simulink model "Hardware_Luo_Converter_with_IGBT"  (R2025a)
settings: Solver=VariableStepAuto  StartTime=0.0  StopTime=1  RelTol=1e-3
libraries: spsSeriesRLCBranchLib x5, spsMeanLib x5, spsCurrentMeasurementLib x2, spsVoltageMeasurementLib x2, spsDCVoltageSourceLib x1, spsDiodeLib x1, spsIGBTDiodeLib x1, sps_lib x1
settings Model: Creator=sanat  LastModifiedBy=sanat

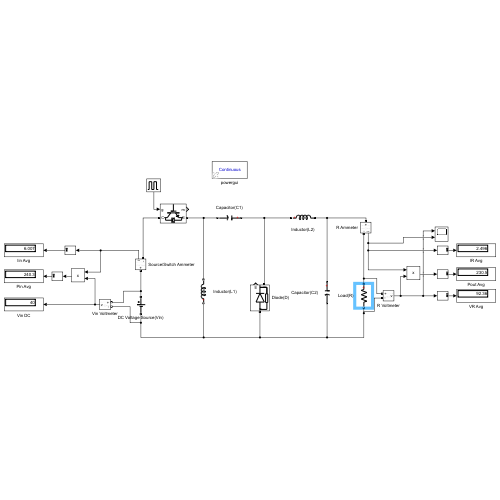
[thumbnail: Simulink's stored preview of the top-level diagram]
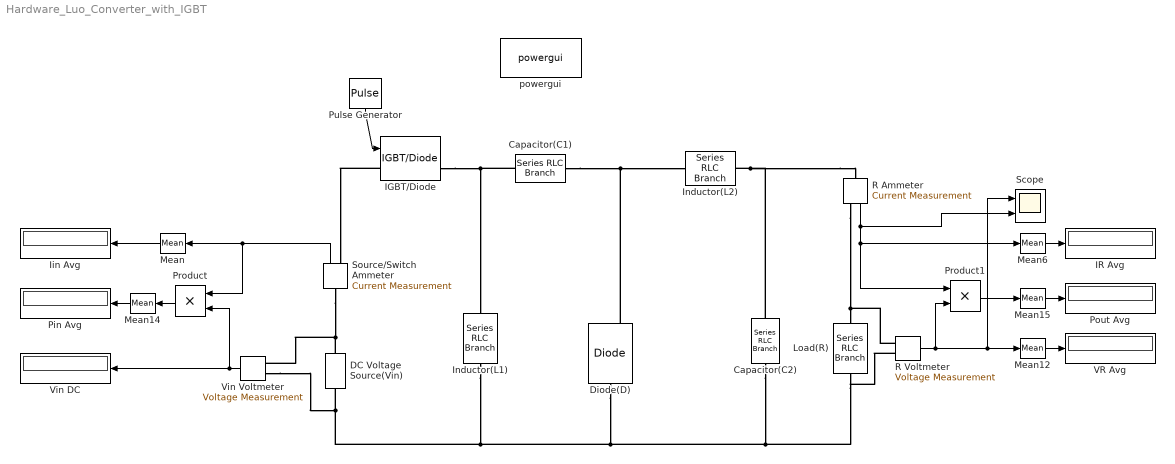
== system Hardware_Luo_Converter_with_IGBT ==
  Capacitor(C1) : spsSeriesRLCBranchLib/Series RLC Branch  LConnTagsString=__new0  RConnTagsString=__new0  BranchType=C  Resistance=1  Inductance=1e-3  SetiL0=off  InitialCurrent=0  Capacitance=470e-6  Setx0=off  InitialVoltage=0  Measurements=None
  Capacitor(C2) : spsSeriesRLCBranchLib/Series RLC Branch  LConnTagsString=__new0  RConnTagsString=__new0  BranchType=C  Resistance=1  Inductance=1e-3  SetiL0=off  InitialCurrent=0  Capacitance=470e-6  Setx0=off  InitialVoltage=0  Measurements=None
  DC Voltage Source(Vin) : spsDCVoltageSourceLib/DC Voltage Source  Amplitude=40  Measurements=None
  Diode(D) : spsDiodeLib/Diode  Ron=0.001  Lon=0  Vf=0.8  IC=0  UseSnubber=0  Rs=500  Cs=250e-9  Measurements=on
  IGBT/Diode : spsIGBTDiodeLib/IGBT//Diode  Ron=1e-2  Rs=1e5  Cs=inf  Measurements=on
  IR Avg : Display
  Iin Avg : Display
  Inductor(L1) : spsSeriesRLCBranchLib/Series RLC Branch  LConnTagsString=__new0  RConnTagsString=__new0  BranchType=L  Resistance=1  Inductance=3.32e-3  SetiL0=off  InitialCurrent=0  Capacitance=1e-6  Setx0=off  InitialVoltage=0  Measurements=None
  Inductor(L2) : spsSeriesRLCBranchLib/Series RLC Branch  LConnTagsString=__new0  RConnTagsString=__new0  BranchType=L  Resistance=1  Inductance=1.52e-3  SetiL0=off  InitialCurrent=0  Capacitance=1e-6  Setx0=off  InitialVoltage=0  Measurements=None
  Load(R) : spsSeriesRLCBranchLib/Series RLC Branch  LConnTagsString=__new0  RConnTagsString=__new0  BranchType=R  Resistance=37  Inductance=1e-3  SetiL0=off  InitialCurrent=0  Capacitance=1e-6  Setx0=off  InitialVoltage=0  Measurements=None
  Mean{,6,12,14..15} (5 alike) : spsMeanLib/Mean  Freq=60  Vinit=0  Ts=0
  Pin Avg : Display
  Pout Avg : Display
  Product : Product
  Product1 : Product
  Pulse Generator : DiscretePulseGenerator  PulseType=Time based  Period=1/20000  PulseWidth=(0.7)*100
  R Ammeter : spsCurrentMeasurementLib/Current Measurement  PhasorSimulation=off  OutputType=Complex  PSBequivalent=0
  R Voltmeter : spsVoltageMeasurementLib/Voltage Measurement  PhasorSimulation=off  OutputType=Complex  PSBequivalent=0
  Scope : Scope  NumInputPorts=2
      settings: ActiveDisplayYMinimum=-126.40513895353823  ActiveDisplayYMaximum=431.16600566715823
  Source/Switch Ammeter : spsCurrentMeasurementLib/Current Measurement  PhasorSimulation=off  OutputType=Complex  PSBequivalent=0
  VR Avg : Display
  Vin DC : Display
  Vin Voltmeter : spsVoltageMeasurementLib/Voltage Measurement  PhasorSimulation=off  OutputType=Complex  PSBequivalent=0
  powergui : sps_lib/powergui  Priority=1  SimulationMode=Continuous  SampleTime=50e-6  frequency=60  Iterations=50  frequencyindice=0  Pbase=100e6  ErrMax=1e-4  UnitsV=kV  UnitsW=MW  buscounter=0  FunctionMessages=off  echomessages=off  EnableUseOfTLC=off  CurrentSourceSwitches=off  DisableSnubberDevices=off  DisableRonSwitches=off  DisableVfSwitches=off  DisplayEquations=off  AutomaticDiscreteSolvers=off  SolverType=Tustin/Backward Euler (TBE)  Interpol=off  ExternalGateDelay=off  methode=off  Ts=100  x0status=blocks  SPID=on  SwTol=0  HookPort=off  NonlinearTolerance=1e-4  nMaxIteration=100  ContinueOnMaxIteration=off  RestoreLinks=warning  ResistiveCurrentMeasurement=off  Frange=[0:2:500]  Ylog=off  Xlog=on  ShowGrid=off  save=off  variable=ZData  structure=0  ZoomFFT=off  StartTime=0.0  cycles=1  DisplayStyle=1  fundamental=60  FreqAxis=off  MaxFrequency=1000  frequencyindicesteady=1  RmsSteady=1  display=off
  wires:
  Pulse Generator/1 -> IGBT/Diode/1
  Vin Voltmeter/1 -> Vin DC/1, Product/2
  Mean/1 -> Iin Avg/1
  Source/Switch Ammeter/1 -> Mean/1, Product/1
  Mean6/1 -> IR Avg/1
  R Ammeter/1 -> Scope/2, Product1/1, Mean6/1
  Mean12/1 -> VR Avg/1
  R Voltmeter/1 -> Scope/1, Mean12/1, Product1/2
  Mean14/1 -> Pin Avg/1
  Product/1 -> Mean14/1
  Mean15/1 -> Pout Avg/1
  Product1/1 -> Mean15/1
  connections:
  DC Voltage Source(Vin)/RConn1 -- Vin Voltmeter/LConn1 -- Source/Switch Ammeter/LConn1
  Capacitor(C1)/RConn1 -- IGBT/Diode/RConn1 -- Inductor(L1)/RConn1
  Inductor(L1)/LConn1 -- R Voltmeter/LConn2 -- Load(R)/RConn1 -- Capacitor(C2)/RConn1 -- Diode(D)/LConn1 -- Vin Voltmeter/LConn2 -- DC Voltage Source(Vin)/LConn1
  Inductor(L2)/RConn1 -- R Ammeter/LConn1 -- Capacitor(C2)/LConn1
  IGBT/Diode/LConn1 -- Source/Switch Ammeter/RConn1
  R Ammeter/RConn1 -- R Voltmeter/LConn1 -- Load(R)/LConn1
  Diode(D)/RConn1 -- Inductor(L2)/LConn1 -- Capacitor(C1)/LConn1
